simulink model "motors"  (R2026a)
settings: Solver=VariableStepAuto
values from neighbouring files (symbols this model uses):
  b_thrust_coeff = 1.5108*10^(-5)    (= 1.5108e-05)    [dz_1_model.m]
  d_grag_factor = 4.406*10*(-7)    (= -308.42)    [dz_1_model.m]
  Ip_inertia = 4.439*10^(-5)    (= 4.439e-05)    [dz_1_model.m]
  lever = 0.124    [dz_1_model.m]
settings Model: Creator=vas77  LastModifiedBy=vas77

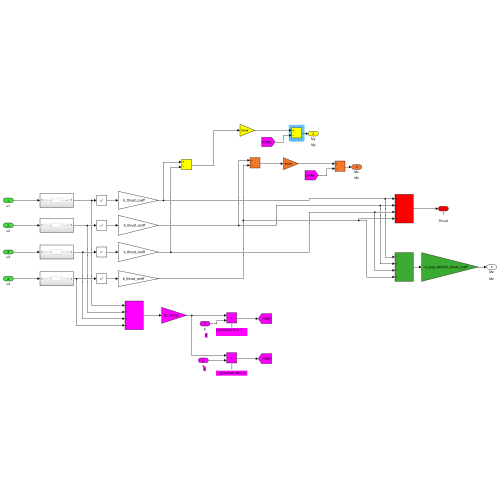
[thumbnail: Simulink's stored preview of the top-level diagram]
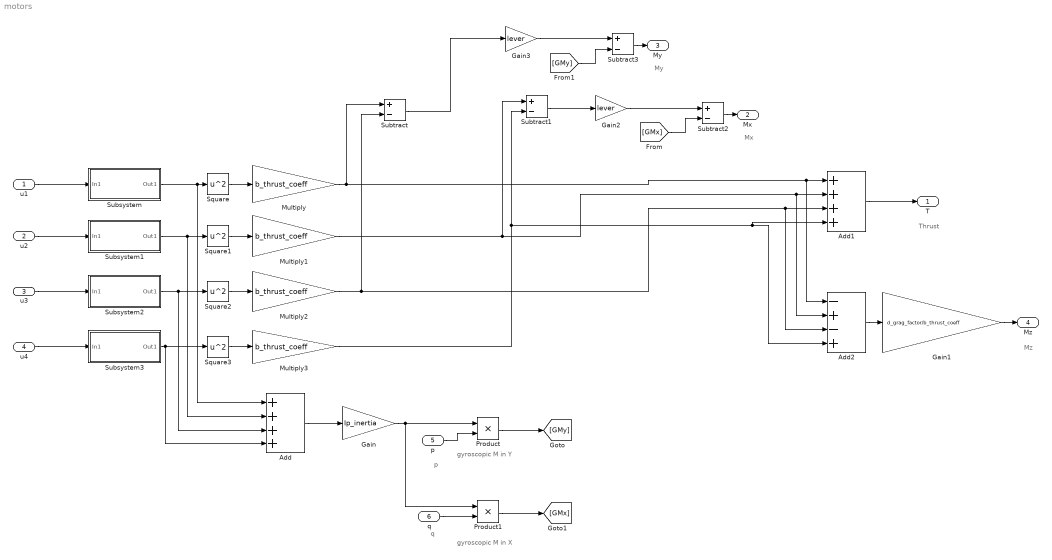
== system motors ==
  note: Mz
  note: Mx
  note: Thrust
  note: q
  note: p
  note: gyroscopic M in Y
  note: gyroscopic M in X
  note: My
  u1 : Inport
  u2 : Inport  Port=2
  u3 : Inport  Port=3
  u4 : Inport  Port=4
  p : Inport  Port=5
  q : Inport  Port=6
  Add : Sum  Inputs=++++
  Add1 : Sum  Inputs=++++
  Add2 : Sum  Inputs=-+-+
  Gain : Gain  Gain=Ip_inertia
  Gain1 : Gain  Gain=d_grag_factor/b_thrust_coeff
  Gain2 : Gain  Gain=lever
  Gain3 : Gain  Gain=lever
  Multiply{,1..3} (4 alike) : Gain  Gain=b_thrust_coeff
  Product : Product
  Product1 : Product
  Square{,1..3} (4 alike) : Math  Operator=square
  Subsystem : Subsystem
  Subsystem1 : Subsystem
  Subsystem2 : Subsystem
  Subsystem3 : Subsystem
  Subtract{,1..3} (4 alike) : Sum  Inputs=+-
  T : Outport
  Mx : Outport  Port=2
  My : Outport  Port=3
  Mz : Outport  Port=4
  wires:
  u1/1 -> Subsystem/1(In1)
  u2/1 -> Subsystem1/1(In1)
  u3/1 -> Subsystem2/1(In1)
  u4/1 -> Subsystem3/1(In1)
  Subsystem1/1(Out1) -> Add/2, Square1/1
  Subsystem/1(Out1) -> Add/1, Square/1
  Subsystem2/1(Out1) -> Add/3, Square2/1
  Subsystem3/1(Out1) -> Add/4, Square3/1
  Square/1 -> Multiply/1
  Square2/1 -> Multiply2/1
  Square3/1 -> Multiply3/1
  Square1/1 -> Multiply1/1
  Add/1 -> Gain/1
  Gain/1 -> Product1/1, Product/1
  p/1 -> Product/2
  q/1 -> Product1/2
  Product/1 -> [GMy]
  Product1/1 -> [GMx]
  Multiply/1 -> Add2/1, Add1/1, Subtract/1
  Multiply1/1 -> Add2/2, Add1/2, Subtract1/1
  Multiply2/1 -> Add2/3, Add1/3, Subtract/2
  Multiply3/1 -> Subtract1/2, Add2/4, Add1/4
  Add2/1 -> Gain1/1
  Add1/1 -> T/1
  Gain2/1 -> Subtract2/1
  Subtract1/1 -> Gain2/1
  [GMx] -> Subtract2/2
  Subtract2/1 -> Mx/1
  Gain3/1 -> Subtract3/1
  [GMy] -> Subtract3/2
  Subtract3/1 -> My/1
  Subtract/1 -> Gain3/1
  Gain1/1 -> Mz/1

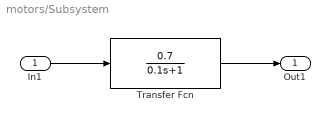
== system motors/Subsystem ==
  In1 : Inport
  Transfer Fcn : TransferFcn  Numerator=[0.7]  Denominator=[0.1 1]
  Out1 : Outport
  wires:
  In1/1 -> Transfer Fcn/1
  Transfer Fcn/1 -> Out1/1

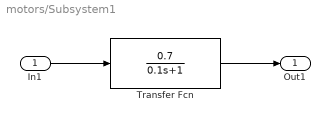
== system motors/Subsystem1 ==
  In1 : Inport
  Transfer Fcn : TransferFcn  Numerator=[0.7]  Denominator=[0.1 1]
  Out1 : Outport
  wires:
  In1/1 -> Transfer Fcn/1
  Transfer Fcn/1 -> Out1/1

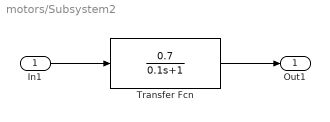
== system motors/Subsystem2 ==
  In1 : Inport
  Transfer Fcn : TransferFcn  Numerator=[0.7]  Denominator=[0.1 1]
  Out1 : Outport
  wires:
  In1/1 -> Transfer Fcn/1
  Transfer Fcn/1 -> Out1/1

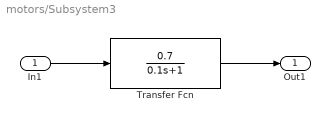
== system motors/Subsystem3 ==
  In1 : Inport
  Transfer Fcn : TransferFcn  Numerator=[0.7]  Denominator=[0.1 1]
  Out1 : Outport
  wires:
  In1/1 -> Transfer Fcn/1
  Transfer Fcn/1 -> Out1/1
